simulink model "EEE_Lab3_CSE21180"  (R2024b)
settings: Solver=VariableStepAuto  StartTime=0.0  StopTime=0.1  RelTol=1e-3
libraries: spsRMSLib x12, spsACVoltageSourceLib x6, spsCurrentMeasurementLib x6, eePowerMeasurement x6, spsSeriesRLCBranchLib x6, spsVoltageMeasurementLib x6, sps_lib x1
settings Model: Creator=LENOVO  LastModifiedBy=surmy

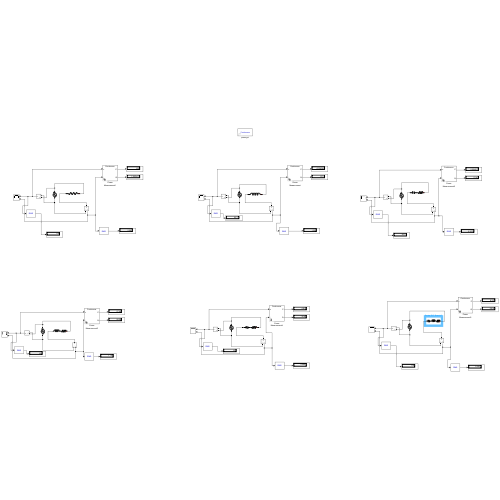
[thumbnail: Simulink's stored preview of the top-level diagram]
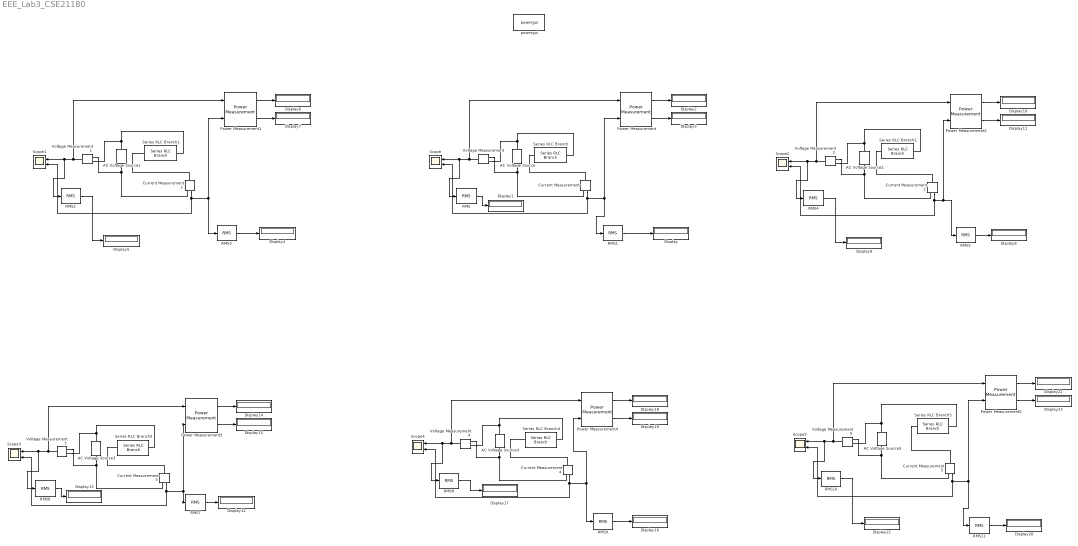
== system EEE_Lab3_CSE21180 ==
  AC Voltage Source : spsACVoltageSourceLib/AC Voltage Source  Amplitude=141.41  Phase=-90  Frequency=50  SampleTime=0  Measurements=None  BusType=swing  Pref=10e3  Qref=0  Qmin=-inf  Qmax=+inf
  AC Voltage Source{1,3..5} (4 alike) : spsACVoltageSourceLib/AC Voltage Source  Amplitude=141.41  Phase=0  Frequency=50  SampleTime=0  Measurements=None  BusType=swing  Pref=10e3  Qref=0  Qmin=-inf  Qmax=+inf
  AC Voltage Source2 : spsACVoltageSourceLib/AC Voltage Source  Amplitude=141.41  Phase=90  Frequency=50  SampleTime=0  Measurements=None  BusType=swing  Pref=10e3  Qref=0  Qmin=-inf  Qmax=+inf
  Current Measurement{,1..5} (6 alike) : spsCurrentMeasurementLib/Current Measurement  PhasorSimulation=off  OutputType=Complex  PSBequivalent=0
  Display{,1..23} (24 alike) : Display
  Power Measurement{,1..5} (6 alike) : eePowerMeasurement/Power Measurement  LabelModeActiveChoice=Continuous  F=50  K=1  Ts=0
  RMS{,1..11} (12 alike) : spsRMSLib/RMS  TrueRMS=on  Freq=60  RMSInit=120  Ts=0
  Scope{,1..5} (6 alike) : Scope  NumInputPorts=2
  Series RLC Branch : spsSeriesRLCBranchLib/Series RLC Branch  LConnTagsString=__new0  RConnTagsString=__new0  BranchType=L  Resistance=50  Inductance=0.25  SetiL0=off  InitialCurrent=0  Capacitance=1e-5  Setx0=off  InitialVoltage=0  Measurements=None
  Series RLC Branch1 : spsSeriesRLCBranchLib/Series RLC Branch  LConnTagsString=__new0  RConnTagsString=__new0  BranchType=R  Resistance=50  Inductance=0.25  SetiL0=off  InitialCurrent=0  Capacitance=1e-5  Setx0=off  InitialVoltage=0  Measurements=None
  Series RLC Branch2 : spsSeriesRLCBranchLib/Series RLC Branch  LConnTagsString=__new0  RConnTagsString=__new0  BranchType=RC  Resistance=0.0001  Inductance=0.25  SetiL0=off  InitialCurrent=0  Capacitance=10e-6  Setx0=off  InitialVoltage=0  Measurements=None
  Series RLC Branch3 : spsSeriesRLCBranchLib/Series RLC Branch  LConnTagsString=__new0  RConnTagsString=__new0  BranchType=RL  Resistance=50  Inductance=0.25  SetiL0=off  InitialCurrent=0  Capacitance=1e-5  Setx0=off  InitialVoltage=0  Measurements=None
  Series RLC Branch4 : spsSeriesRLCBranchLib/Series RLC Branch  LConnTagsString=__new0  RConnTagsString=__new0  BranchType=RC  Resistance=50  Inductance=0.25  SetiL0=off  InitialCurrent=0  Capacitance=10e-6  Setx0=off  InitialVoltage=0  Measurements=None
  Series RLC Branch5 : spsSeriesRLCBranchLib/Series RLC Branch  LConnTagsString=__new0  RConnTagsString=__new0  BranchType=RLC  Resistance=50  Inductance=0.25  SetiL0=off  InitialCurrent=0  Capacitance=10e-6  Setx0=off  InitialVoltage=0  Measurements=None
  Voltage Measurement{,1..5} (6 alike) : spsVoltageMeasurementLib/Voltage Measurement  PhasorSimulation=off  OutputType=Complex  PSBequivalent=0
  powergui : sps_lib/powergui  Priority=1  SimulationMode=Continuous  SampleTime=50e-6  frequency=60  Iterations=50  frequencyindice=50  Pbase=100e6  ErrMax=1e-4  UnitsV=kV  UnitsW=MW  buscounter=0  FunctionMessages=off  echomessages=off  EnableUseOfTLC=off  CurrentSourceSwitches=off  DisableSnubberDevices=off  DisableRonSwitches=off  DisableVfSwitches=off  DisplayEquations=off  AutomaticDiscreteSolvers=off  SolverType=Tustin/Backward Euler (TBE)  Interpol=off  ExternalGateDelay=off  methode=off  Ts=100  x0status=blocks  SPID=on  SwTol=0  HookPort=off  NonlinearTolerance=1e-4  nMaxIteration=100  ContinueOnMaxIteration=off  RestoreLinks=warning  ResistiveCurrentMeasurement=off  Frange=[0:2:500]  Ylog=off  Xlog=on  ShowGrid=off  save=off  variable=ZData  structure=0  ZoomFFT=off  StartTime=0.0  cycles=1  DisplayStyle=1  fundamental=60  FreqAxis=off  MaxFrequency=1000  frequencyindicesteady=1  RmsSteady=1  display=off
  wires:
  RMS1/1 -> Display/1
  Voltage Measurement/1 -> Power Measurement/1, RMS/1, Scope/1
  Current Measurement/1 -> Power Measurement/2, RMS1/1, Scope/2
  RMS/1 -> Display1/1
  Power Measurement/1 -> Display2/1
  Power Measurement/2 -> Display3/1
  Power Measurement1/1 -> Display6/1
  Power Measurement1/2 -> Display7/1
  RMS3/1 -> Display4/1
  RMS2/1 -> Display5/1
  Current Measurement1/1 -> Power Measurement1/2, RMS3/1, Scope1/2
  Voltage Measurement1/1 -> Power Measurement1/1, RMS2/1, Scope1/1
  Power Measurement2/1 -> Display10/1
  Power Measurement2/2 -> Display11/1
  RMS5/1 -> Display8/1
  RMS4/1 -> Display9/1
  Current Measurement2/1 -> RMS5/1, Power Measurement2/2, Scope2/2
  Voltage Measurement2/1 -> Power Measurement2/1, RMS4/1, Scope2/1
  Current Measurement3/1 -> Power Measurement3/2, RMS7/1, Scope3/2
  Voltage Measurement3/1 -> Power Measurement3/1, RMS6/1, Scope3/1
  RMS6/1 -> Display13/1
  RMS7/1 -> Display12/1
  Power Measurement3/2 -> Display15/1
  Power Measurement3/1 -> Display14/1
  Current Measurement4/1 -> Power Measurement4/2, RMS9/1, Scope4/2
  Voltage Measurement4/1 -> Power Measurement4/1, RMS8/1, Scope4/1
  RMS8/1 -> Display17/1
  RMS9/1 -> Display16/1
  Power Measurement4/2 -> Display19/1
  Power Measurement4/1 -> Display18/1
  Current Measurement5/1 -> Power Measurement5/2, RMS11/1, Scope5/2
  Voltage Measurement5/1 -> Power Measurement5/1, RMS10/1, Scope5/1
  RMS10/1 -> Display21/1
  RMS11/1 -> Display20/1
  Power Measurement5/2 -> Display23/1
  Power Measurement5/1 -> Display22/1
  connections:
  AC Voltage Source/RConn1 -- Voltage Measurement/LConn1 -- Series RLC Branch/LConn1
  AC Voltage Source/LConn1 -- Voltage Measurement/LConn2 -- Current Measurement/RConn1
  Current Measurement/LConn1 -- Series RLC Branch/RConn1
  AC Voltage Source1/RConn1 -- Voltage Measurement1/LConn1 -- Series RLC Branch1/LConn1
  AC Voltage Source1/LConn1 -- Voltage Measurement1/LConn2 -- Current Measurement1/RConn1
  Current Measurement1/LConn1 -- Series RLC Branch1/RConn1
  AC Voltage Source2/RConn1 -- Voltage Measurement2/LConn1 -- Series RLC Branch2/LConn1
  AC Voltage Source2/LConn1 -- Voltage Measurement2/LConn2 -- Current Measurement2/RConn1
  Current Measurement2/LConn1 -- Series RLC Branch2/RConn1
  AC Voltage Source3/LConn1 -- Voltage Measurement3/LConn2 -- Current Measurement3/RConn1
  AC Voltage Source3/RConn1 -- Voltage Measurement3/LConn1 -- Series RLC Branch3/LConn1
  Current Measurement3/LConn1 -- Series RLC Branch3/RConn1
  AC Voltage Source4/LConn1 -- Voltage Measurement4/LConn2 -- Current Measurement4/RConn1
  AC Voltage Source4/RConn1 -- Voltage Measurement4/LConn1 -- Series RLC Branch4/LConn1
  Current Measurement4/LConn1 -- Series RLC Branch4/RConn1
  AC Voltage Source5/LConn1 -- Voltage Measurement5/LConn2 -- Current Measurement5/RConn1
  AC Voltage Source5/RConn1 -- Voltage Measurement5/LConn1 -- Series RLC Branch5/LConn1
  Current Measurement5/LConn1 -- Series RLC Branch5/RConn1
